simulink model "UR5"  (R2024b)
settings: Solver=FixedStepAuto  StartTime=0.0  StopTime=10.0  FixedStep=0.01  RelTol=1e-3
values from neighbouring files (symbols this model uses):
  a1 = 0.0    (= 0)    [UR5_param.m]
  a2 = -0.425    [UR5_param.m]
  a3 = -0.3925    [UR5_param.m]
  a4 = 0.0    (= 0)    [UR5_param.m]
  a5 = 0.0    (= 0)    [UR5_param.m]
  a6 = 0.0    (= 0)    [UR5_param.m]
  a_vec = [a1, a2, a3, a4, a5, a6]    [UR5_param.m]
  alpha1 = pi/2    (= 1.57079632679)    [UR5_param.m]
  alpha2 = 0.0    (= 0)    [UR5_param.m]
  alpha3 = 0.0    (= 0)    [UR5_param.m]
  alpha4 = pi/2    (= 1.57079632679)    [UR5_param.m]
  alpha5 = -pi/2    (= -1.57079632679)    [UR5_param.m]
  alpha6 = 0.0    (= 0)    [UR5_param.m]
  alpha_vec = [alpha1, alpha2, alpha3, alpha4, alpha5, alpha6]    [UR5_param.m]
  d1 = 0.08916    [UR5_param.m]
  d2 = 0.0    (= 0)    [UR5_param.m]
  d3 = 0.0    (= 0)    [UR5_param.m]
  d4 = 0.10915    [UR5_param.m]
  d5 = 0.09465    [UR5_param.m]
  d6 = 0.0823    [UR5_param.m]
  d_vec = [d1, d2, d3, d4, d5, d6]    [UR5_param.m]
  dtheta_initial_vec = [0, 0, 0.04, 0, 0, 0]    [UR5_param.m]
  inertiaArray = zeros(3, 3, 6)    [UR5_param.m]
  masses = [3.7, 8.393, 2.275, 1.219, 1.219, 0.1879]    [UR5_param.m]
  theta_initial_vec = [0.3, 0.2, 0, 0, 0, 0]    [UR5_param.m]
libraries: robotmaniplib x2
settings Model: Creator=zhes  LastModifiedBy=zhes

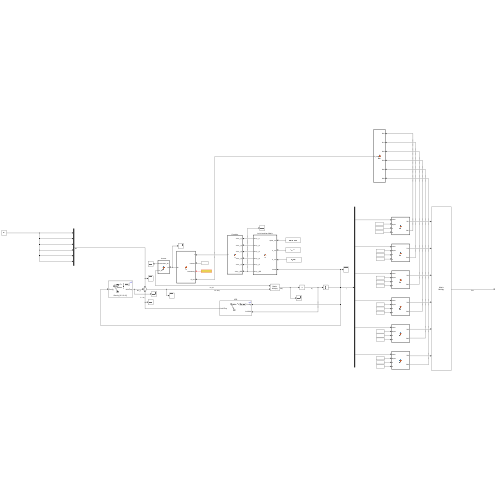
[thumbnail: Simulink's stored preview of the top-level diagram]
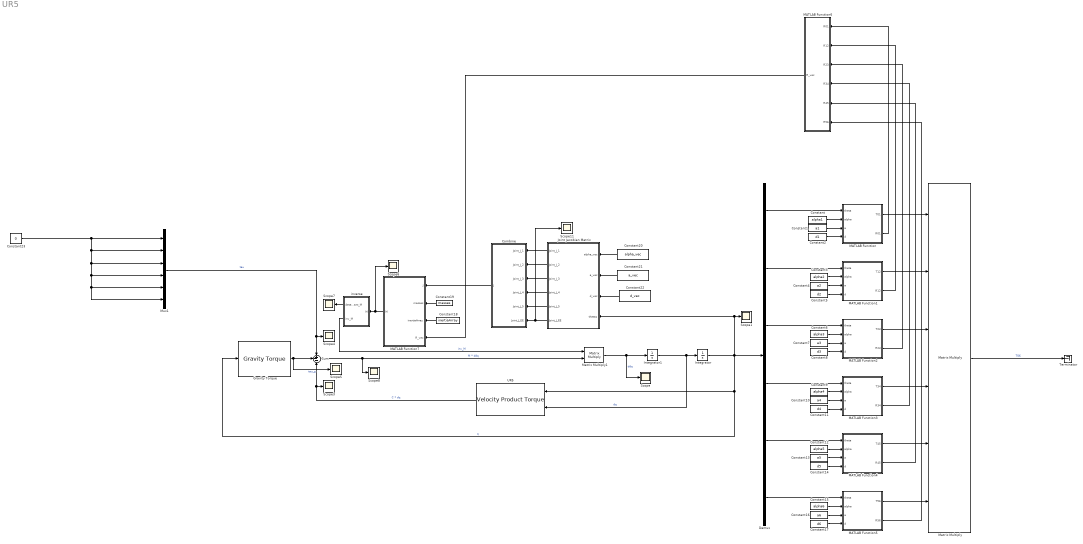
== system UR5 ==
  Combine : MATLAB Function  TreatAsAtomicUnit=on
  Constant : Constant  Value=alpha1
  Constant1 : Constant  Value=a1
  Constant10 : Constant  Value=a4
  Constant11 : Constant  Value=d4
  Constant12 : Constant  Value=alpha5
  Constant13 : Constant  Value=a5
  Constant14 : Constant  Value=d5
  Constant15 : Constant  Value=alpha6
  Constant16 : Constant  Value=a6
  Constant17 : Constant  Value=d6
  Constant18 : Constant  Value=inertiaArray
  Constant19 : Constant  Value=masses
  Constant2 : Constant  Value=d1
  Constant20 : Constant  Value=alpha_vec
  Constant21 : Constant  Value=a_vec
  Constant22 : Constant  Value=d_vec
  Constant23 : Constant  Value=0
  Constant3 : Constant  Value=alpha2
  Constant4 : Constant  Value=a2
  Constant5 : Constant  Value=d2
  Constant6 : Constant  Value=alpha3
  Constant7 : Constant  Value=a3
  Constant8 : Constant  Value=d3
  Constant9 : Constant  Value=alpha4
  Demux : Demux  Outputs=6
  Gravity Torque : robotmaniplib/Gravity Torque  RigidBodyTree=ur5  SimulateUsing=Interpreted execution
  Integrator : Integrator  InitialCondition=theta_initial_vec
  Integrator1 : Integrator  InitialCondition=dtheta_initial_vec
  Joint Jacobian Matrix : MATLAB Function  TreatAsAtomicUnit=on
  MATLAB Function : MATLAB Function  TreatAsAtomicUnit=on
  MATLAB Function1 : MATLAB Function  TreatAsAtomicUnit=on
  MATLAB Function2 : MATLAB Function  TreatAsAtomicUnit=on
  MATLAB Function3 : MATLAB Function  TreatAsAtomicUnit=on
  MATLAB Function4 : MATLAB Function  TreatAsAtomicUnit=on
  MATLAB Function5 : MATLAB Function  TreatAsAtomicUnit=on
  MATLAB Function6 : MATLAB Function  TreatAsAtomicUnit=on
  MATLAB Function7 : MATLAB Function  TreatAsAtomicUnit=on
  Matrix Multiply : Product  Inputs=6  Multiplication=Matrix(*)
  Matrix Multiply1 : Product  Multiplication=Matrix(*)
  Mux1 : Mux  Inputs=6
  Scope{,1,3..8,11} (9 alike) : Scope
  Sum : Sum  Inputs=+--
  Terminator : Terminator
  UR5 : robotmaniplib/Velocity Product Torque  RigidBodyTree=ur5  SimulateUsing=Interpreted execution
  inverse : MATLAB Function  TreatAsAtomicUnit=on
  wires:
  MATLAB Function/1(T01) -> Matrix Multiply/1
  MATLAB Function1/1(T12) -> Matrix Multiply/2
  MATLAB Function2/1(T23) -> Matrix Multiply/3
  MATLAB Function3/1(T34) -> Matrix Multiply/4
  MATLAB Function4/1(T45) -> Matrix Multiply/5
  MATLAB Function5/1(T56) -> Matrix Multiply/6
  Matrix Multiply/1 -> Terminator/1  "T06"
  Constant/1 -> MATLAB Function/2(alpha)
  Constant1/1 -> MATLAB Function/3(a)
  Constant2/1 -> MATLAB Function/4(d)
  Constant3/1 -> MATLAB Function1/2(alpha)
  Constant5/1 -> MATLAB Function1/4(d)
  Constant4/1 -> MATLAB Function1/3(a)
  Constant8/1 -> MATLAB Function2/4(d)
  Constant6/1 -> MATLAB Function2/2(alpha)
  Constant7/1 -> MATLAB Function2/3(a)
  Constant11/1 -> MATLAB Function3/4(d)
  Constant9/1 -> MATLAB Function3/2(alpha)
  Constant10/1 -> MATLAB Function3/3(a)
  Constant14/1 -> MATLAB Function4/4(d)
  Constant12/1 -> MATLAB Function4/2(alpha)
  Constant13/1 -> MATLAB Function4/3(a)
  Constant17/1 -> MATLAB Function5/4(d)
  Constant15/1 -> MATLAB Function5/2(alpha)
  Constant16/1 -> MATLAB Function5/3(a)
  Integrator1/1 -> UR5/2, Integrator/1  "dq"
  Integrator/1 -> Joint Jacobian Matrix/4(thetas), Scope1/1, Gravity Torque/1, UR5/1, Demux/1  "q"
  Demux/6 -> MATLAB Function5/1(theta)
  Demux/5 -> MATLAB Function4/1(theta)
  Demux/4 -> MATLAB Function3/1(theta)
  Demux/3 -> MATLAB Function2/1(theta)
  Demux/2 -> MATLAB Function1/1(theta)
  Demux/1 -> MATLAB Function/1(theta)
  Matrix Multiply1/1 -> Scope/1, Integrator1/1  "ddq"
  Sum/1 -> Matrix Multiply1/2, Scope8/1  "M * ddq"
  Gravity Torque/1 -> Scope5/1, Sum/2  "tau_g"
  UR5/1 -> Scope3/1, Sum/3  "C * dq"
  Joint Jacobian Matrix/1(Joint_J_1) -> Combine/1(Joint_J_1)
  Joint Jacobian Matrix/2(Joint_J_2) -> Combine/2(Joint_J_2)
  Joint Jacobian Matrix/6(Joint_J_EE) -> Scope11/1, Combine/6(Joint_J_EE)
  Joint Jacobian Matrix/5(Joint_J_5) -> Combine/5(Joint_J_5)
  Joint Jacobian Matrix/4(Joint_J_4) -> Combine/4(Joint_J_4)
  Joint Jacobian Matrix/3(Joint_J_3) -> Combine/3(Joint_J_3)
  Combine/1(J) -> MATLAB Function7/1(J)
  Constant19/1 -> MATLAB Function7/2(masses)
  Mux1/1 -> Scope4/1, Sum/1  "tau"
  MATLAB Function7/1(M) -> Scope6/1, inverse/1(M)
  inverse/2(inv_M) -> Matrix Multiply1/1  "inv_M"
  Constant20/1 -> Joint Jacobian Matrix/1(alpha_vec)
  Constant21/1 -> Joint Jacobian Matrix/2(a_vec)
  Constant22/1 -> Joint Jacobian Matrix/3(d_vec)
  Constant18/1 -> MATLAB Function7/3(inertiaArray)
  MATLAB Function/2(R01) -> MATLAB Function6/1(R01)
  MATLAB Function1/2(R12) -> MATLAB Function6/2(R12)
  MATLAB Function2/2(R23) -> MATLAB Function6/3(R23)
  MATLAB Function3/2(R34) -> MATLAB Function6/4(R34)
  MATLAB Function4/2(R45) -> MATLAB Function6/5(R45)
  MATLAB Function5/2(R56) -> MATLAB Function6/6(R56)
  MATLAB Function6/1(R_vec) -> MATLAB Function7/4(R_vec)
  inverse/1(determinant_M) -> Scope7/1
  Constant23/1 -> Mux1/6, Mux1/5, Mux1/4, Mux1/3, Mux1/2, Mux1/1

== matlab function UR5/MATLAB Function7 ==
  data: J input; M output; masses input; inertiaArray input; R_vec input
function M = fcn(J, masses, inertiaArray, R_vec)

J1 = J(:,:,1); 
J2 = J(:,:,2);
J3 = J(:,:,3); 
J4 = J(:,:,4);
J5 = J(:,:,5);
J6 = J(:,:,6);

Jv1 = J1(1:3, :);
Jw1 = J1(4:6, :);

Jv2 = J2(1:3, :);
Jw2 = J2(4:6, :);

Jv3 = J3(1:3, :);
Jw3 = J3(4:6, :);

Jv4 = J4(1:3, :);
Jw4 = J4(4:6, :);

Jv5 = J5(1:3, :);
Jw5 = J5(4:6, :);

Jv6 = J6(1:3, :);
Jw6 = J6(4:6, :);

M = masses(1) * Jv1.' * Jv1 + ...
    masses(2) * Jv2.' * Jv2 + ...
    masses(3) * Jv3.' * Jv3 + ...
    masses(4) * Jv4.' * Jv4 + ...
    masses(5) * Jv5.' * Jv5 + ...
    masses(6) * Jv6.' * Jv6 + ...
    Jw1.' * R_vec(:,:,1) * inertiaArray(:,:,1) * R_vec(:,:,1).' * Jw1 + ...
    Jw2.' * R_vec(:,:,2) * inertiaArray(:,:,2) * R_vec(:,:,2).' * Jw2 + ...
    Jw3.' * R_vec(:,:,3) * inertiaArray(:,:,3) * R_vec(:,:,3).' * Jw3 + ...
    Jw4.' * R_vec(:,:,4) * inertiaArray(:,:,4) * R_vec(:,:,4).' * Jw4 + ...
    Jw5.' * R_vec(:,:,5) * inertiaArray(:,:,5) * R_vec(:,:,5).' * Jw5 + ...
    Jw6.' * R_vec(:,:,6) * inertiaArray(:,:,6) * R_vec(:,:,6).' * Jw6;

end

== matlab function UR5/Combine ==
  data: Joint_J_1 input; J output; Joint_J_2 input; Joint_J_3 input; Joint_J_4 input; Joint_J_5 input; Joint_J_EE input
function J = fcn(Joint_J_1, Joint_J_2, Joint_J_3, Joint_J_4, Joint_J_5, Joint_J_EE)

J = zeros(6,6,6);
J(:,:,1) = Joint_J_1;
J(:,:,2) = Joint_J_2;
J(:,:,3) = Joint_J_3;
J(:,:,4) = Joint_J_4;
J(:,:,5) = Joint_J_5;
J(:,:,6) = Joint_J_EE;

== matlab function UR5/MATLAB Function6 ==
  data: R01 input; R_vec output; R12 input; R23 input; R34 input; R45 input; R56 input
function R_vec = fcn(R01, R12, R23, R34, R45, R56)

R_vec = zeros(3,3,6);

R_vec(:,:,1) = R01;
R_vec(:,:,2) = R12;
R_vec(:,:,3) = R23;
R_vec(:,:,4) = R34;
R_vec(:,:,5) = R45;
R_vec(:,:,6) = R56;

== matlab function UR5/MATLAB Function1 ==
  data: theta input; T12 output; alpha input; a input; d input; R12 output
function [T12, R12]= fcn(theta,alpha,a,d)

T12 = [ cos(theta),  -sin(theta) * cos(alpha),   sin(theta) * sin(alpha),  a * cos(theta);
        sin(theta),   cos(theta) * cos(alpha),  -cos(theta) * sin(alpha),  a * sin(theta);
                 0,                sin(alpha),                cos(alpha),               d;
                 0,                         0,                         0,               1];

R12 = T12(1:3,1:3);

== matlab function UR5/MATLAB Function ==
  data: theta input; T01 output; alpha input; a input; d input; R01 output
function [T01, R01]= fcn(theta,alpha,a,d)

T01 = [ cos(theta),  -sin(theta) * cos(alpha),   sin(theta) * sin(alpha),  a * cos(theta);
        sin(theta),   cos(theta) * cos(alpha),  -cos(theta) * sin(alpha),  a * sin(theta);
                 0,                sin(alpha),                cos(alpha),               d;
                 0,                         0,                         0,               1];

R01 = T01(1:3,1:3);

== matlab function UR5/MATLAB Function2 ==
  data: theta input; T23 output; alpha input; a input; d input; R23 output
function [T23, R23]= fcn(theta,alpha,a,d)

T23 = [ cos(theta),  -sin(theta) * cos(alpha),   sin(theta) * sin(alpha),  a * cos(theta);
        sin(theta),   cos(theta) * cos(alpha),  -cos(theta) * sin(alpha),  a * sin(theta);
                 0,                sin(alpha),                cos(alpha),               d;
                 0,                         0,                         0,               1];

R23 = T23(1:3,1:3);

== matlab function UR5/MATLAB Function3 ==
  data: theta input; T34 output; alpha input; a input; d input; R34 output
function [T34, R34]= fcn(theta,alpha,a,d)

T34 = [ cos(theta),  -sin(theta) * cos(alpha),   sin(theta) * sin(alpha),  a * cos(theta);
        sin(theta),   cos(theta) * cos(alpha),  -cos(theta) * sin(alpha),  a * sin(theta);
                 0,                sin(alpha),                cos(alpha),               d;
                 0,                         0,                         0,               1];

R34 = T34(1:3,1:3);

== matlab function UR5/MATLAB Function4 ==
  data: theta input; T45 output; alpha input; a input; d input; R45 output
function [T45, R45]= fcn(theta,alpha,a,d)

T45 = [ cos(theta),  -sin(theta) * cos(alpha),   sin(theta) * sin(alpha),  a * cos(theta);
        sin(theta),   cos(theta) * cos(alpha),  -cos(theta) * sin(alpha),  a * sin(theta);
                 0,                sin(alpha),                cos(alpha),               d;
                 0,                         0,                         0,               1];

R45 = T45(1:3,1:3);

== matlab function UR5/MATLAB Function5 ==
  data: theta input; T56 output; alpha input; a input; d input; R56 output
function [T56, R56]= fcn(theta,alpha,a,d)

T56 = [ cos(theta),  -sin(theta) * cos(alpha),   sin(theta) * sin(alpha),  a * cos(theta);
        sin(theta),   cos(theta) * cos(alpha),  -cos(theta) * sin(alpha),  a * sin(theta);
                 0,                sin(alpha),                cos(alpha),               d;
                 0,                         0,                         0,               1];

R56 = T56(1:3,1:3);

== matlab function UR5/Joint Jacobian Matrix ==
  data: alpha_vec input; a_vec input; d_vec input; Joint_J_1 output; Joint_J_2 output; Joint_J_3 output; Joint_J_4 output; Joint_J_5 output; thetas input; Joint_J_EE output
function [Joint_J_1, Joint_J_2, Joint_J_3, Joint_J_4, Joint_J_5, Joint_J_EE]= fcn(alpha_vec, a_vec, d_vec, thetas)

% DH parameters: [theta, d, a, alpha]
Joint_DH_params = [
    thetas(1), d_vec(1), a_vec(1), alpha_vec(1);
    thetas(2), d_vec(2), a_vec(2), alpha_vec(2);
    thetas(3), d_vec(3), a_vec(3), alpha_vec(3);
    thetas(4), d_vec(4), a_vec(4), alpha_vec(4);
    thetas(5), d_vec(5), a_vec(5), alpha_vec(5);
    thetas(6), d_vec(6), a_vec(6), alpha_vec(6)
];

Joint_J_EE = UR5_Jacobian(Joint_DH_params, 6, 6); % Joint Jacobian

Joint_J_1 = UR5_Jacobian(Joint_DH_params, 6, 1);
Joint_J_2 = UR5_Jacobian(Joint_DH_params, 6, 2);
Joint_J_3 = UR5_Jacobian(Joint_DH_params, 6, 3);
Joint_J_4 = UR5_Jacobian(Joint_DH_params, 6, 4);
Joint_J_5 = UR5_Jacobian(Joint_DH_params, 6, 5);


    function J = UR5_Jacobian(DH_params, n_joints, n)

        T = eye(4); % Initialize transformation matrix
        Z = zeros(3, n+1); % Store Z vectors (rotation axes)
        P = zeros(3, n+1); % Store P vectors (positions)
    
        % Initialize base frame
        Z(:, 1) = [0; 0; 1]; % Z0 is along z-axis
        P(:, 1) = [0; 0; 0]; % Origin O0
    
        % Forward Kinematics: Calculate each transformation matrix
        for i = 1:n
            theta = DH_params(i, 1);
            d = DH_params(i, 2);
            a = DH_params(i, 3);
            alpha = DH_params(i, 4);
    
            % Transformation matrix using DH parameters
            Ti = [
                cos(theta), -sin(theta)*cos(alpha),  sin(theta)*sin(alpha), a*cos(theta);
                sin(theta),  cos(theta)*cos(alpha), -cos(theta)*sin(alpha), a*sin(theta);
                         0,             sin(alpha),             cos(alpha),            d;
                         0,                      0,                      0,            1
            ];
        
            % Accumulate transformation
            T = T * Ti;
        
            % Store rotation axis and origin
            Z(:, i+1) = T(1:3, 3); % Zi
            P(:, i+1) = T(1:3, 4); % Oi
        end
    
    
        % Jacobian Calculation
        J = zeros(6, n_joints);
        P_i = P(:, end); % joint of interest position
    
        for i = 1:n
            % Linear velocity part
            J(1:3, i) = cross(Z(:, i), P_i - P(:, i));
            % Angular velocity part
            J(4:6, i) = Z(:, i);
        end
    end

end

== matlab function UR5/inverse ==
  data: determinant_M output; M input; inv_M output
function [determinant_M, inv_M]= fcn(M)

determinant_M = det(M);
inv_M = inv(M);
